simulink model "combined_1023"  (R2023a)
settings: Solver=ode45  StartTime=0  StopTime=20  FixedStep=0.001  RelTol=1e-3  AbsTol=1e-6
libraries: simulink x26, dspsigops x4, Solver_SF x1, slpidlib x1
settings Model: ExtModeTrigMode=oneshot  Creator=jhu  LastModifiedBy=Student
settings SolverCC: AutoScaleAbsTol=off  AlgebraicLoopSolver=TrustRegion
settings DataIOCC: SaveFormat=Array  SignalLoggingSaveFormat=ModelDataLogs  ReturnWorkspaceOutputs=off  SignalLoggingName=sigsOut
settings OptimizationCC: BlockReduction=off  BooleanDataType=off  ExpressionDepthLimit=2147483647  LifeSpan=inf
settings DebuggingCC: SaveWithParameterizedLinksMsg=none  UnderspecifiedInitializationDetection=Classic  MergeDetectMultiDrivingBlocksExec=none  SignalResolutionControl=TryResolveAllWithWarning  MultiTaskDSMMsg=warning  MultiTaskCondExecSysMsg=none  FcnCallInpInsideContextMsg=warning  UnconnectedInputMsg=warning  UnconnectedOutputMsg=warning  UnconnectedLineMsg=warning  StateNameClashWarn=warning  SFUnexpectedBacktrackingDiag=warning  SFNoUnconditionalDefaultTransitionDiag=warning  SFExecutionAtInitializationDiag=none  ArithmeticOperatorsInVariantConditions=warning
settings HardwareCC: ProdBitPerPointer=32  ProdBitPerSizeT=32  ProdBitPerPtrDiffT=32  ProdLargestAtomicFloat=None  ProdIntDivRoundTo=Undefined  ProdEndianess=Unspecified  ProdWordSize=32  ProdHWDeviceType=32-bit Generic  TargetUnknown=on
settings ModelReferenceCC: PropagateSignalLabelsOutOfModel=off
settings SFSimCC: SimUseLocalCustomCode=off  CustomCodeUndefinedFunction=UseInterfaceOnly
settings RTWCC: TemplateMakefile=grt_vc.tmf  RTWUseLocalCustomCode=off
settings CodeAppCC: StateflowObjectComments=on
settings GRTTargetCC: TargetFcnLib=ansi_tfl_tmw.mat  TargetLangStandard=C89/C90 (ANSI)  CombineOutputUpdateFcns=off  GRTInterface=on
settings ConfigComp: CovMetricSettings=dw  CovSaveCumulativeToWorkspaceVar=on  CovSaveSingleToWorkspaceVar=on  CovExternalEMLEnable=off

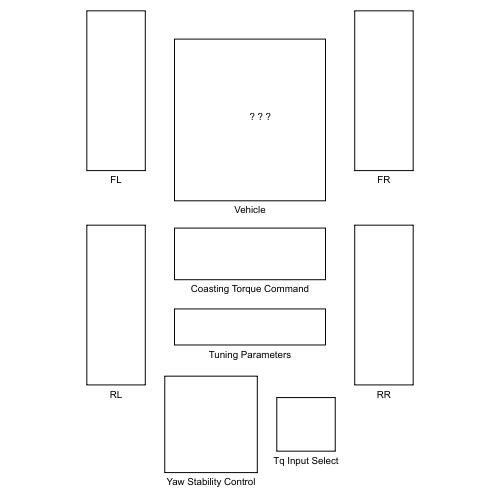
[thumbnail: Simulink's stored preview of the top-level diagram]
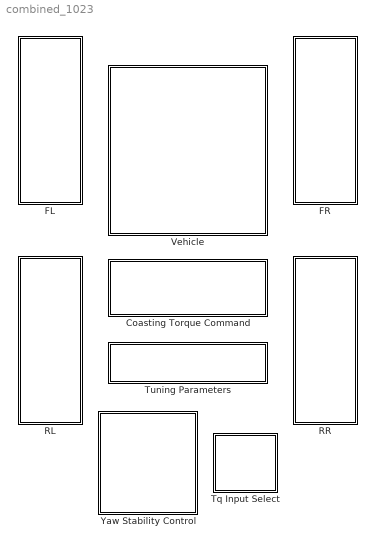
== system combined_1023 ==
  Coasting Torque Command : Subsystem
  FL : Subsystem
  FR : Subsystem
  RL : Subsystem
  RR : Subsystem
  Tq Input Select : Subsystem
  Tuning Parameters : Subsystem
  Vehicle : Subsystem
      mask Display: image('C:\Users\USER\Downloads\vehicle_icon.png'); % Use "Edit Image" on toolstrip to change.
  Yaw Stability Control : Subsystem

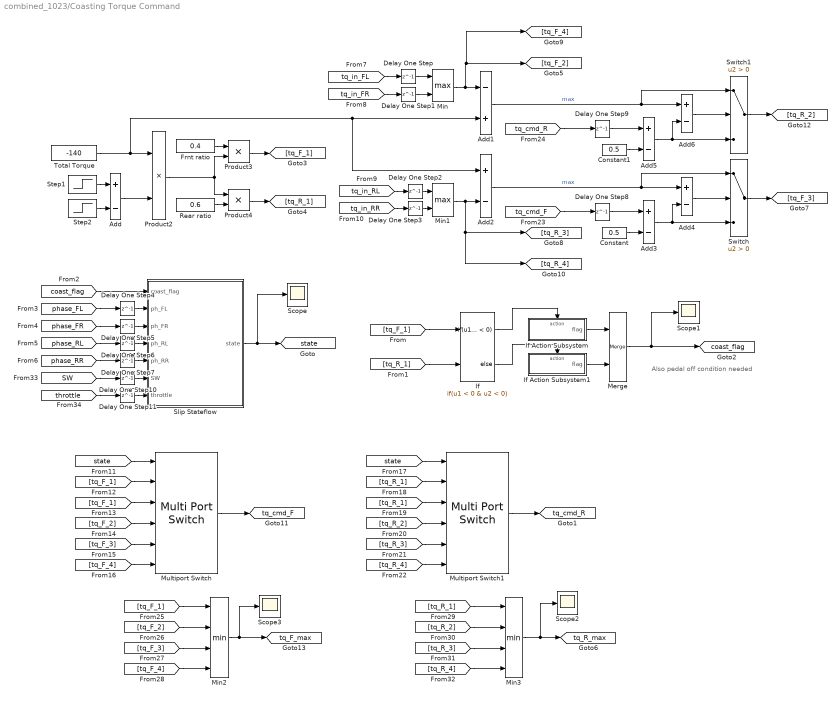
== system combined_1023/Coasting Torque Command ==
  note: Also pedal off condition needed
  Add{,2..6} (6 alike) : Sum  Inputs=+-
  Add1 : Sum  Inputs=-+
  Constant : Constant  Value=0.5
  Constant1 : Constant  Value=0.5
  Delay One Step{,1..7,10..11} (10 alike) : Delay  DelayLength=1
  Delay One Step8 : Delay  DelayLength=1  SampleTime=0.01
  Delay One Step9 : Delay  DelayLength=1  SampleTime=0.01
  Frnt ratio : Constant  Value=0.4  SampleTime=0.01
  If : If  NumInputs=2  IfExpression=u1 < 0 & u2 < 0
  If Action Subsystem : Subsystem  TreatAsAtomicUnit=on
  If Action Subsystem1 : Subsystem  TreatAsAtomicUnit=on
  Merge : Merge
  Min : MinMax  Function=max  Inputs=2
  Min1 : MinMax  Function=max  Inputs=2
  Min2 : MinMax  Inputs=4
  Min3 : MinMax  Inputs=4
  Multiport Switch : MultiPortSwitch  DataPortOrder=Zero-based contiguous  Inputs=5  zeroidx=on  SaturateOnIntegerOverflow=off  InputSameDT=off
  Multiport Switch1 : MultiPortSwitch  DataPortOrder=Zero-based contiguous  Inputs=5  zeroidx=on  SaturateOnIntegerOverflow=off  InputSameDT=off
  Product2 : Product
  Product3 : Product
  Product4 : Product
  Rear ratio : Constant  Value=0.6  SampleTime=0.01
  Scope{,1..3} (4 alike) : Scope
  Slip Stateflow : Stateflow chart  TreatAsAtomicUnit=on
  Step1 : Step  Time=5  SampleTime=0.01
  Step2 : Step  Time=20  SampleTime=0.01
  Switch : Switch  Criteria=u2 > Threshold  SaturateOnIntegerOverflow=off  InputSameDT=off
  Switch1 : Switch  Criteria=u2 > Threshold  SaturateOnIntegerOverflow=off  InputSameDT=off
  Total Torque : Constant  Value=-140  SampleTime=0.01
  tag scope: coast_flag=global, state=global, tq_F_max=global, tq_R_max=global, tq_cmd_F=global, tq_cmd_R=global
  wires:
  [tq_F_1] -> If/1
  [tq_R_1] -> If/2
  If/1 -> If Action Subsystem/Action
  If Action Subsystem/1(flag) -> Merge/1
  If Action Subsystem1/1(flag) -> Merge/2
  If/2 -> If Action Subsystem1/Action
  Merge/1 -> Scope1/1, [coast_flag]
  [coast_flag] -> Slip Stateflow/1(coast_flag)
  [phase_FL] -> Delay One Step4/1
  [phase_FR] -> Delay One Step5/1
  [phase_RL] -> Delay One Step6/1
  [phase_RR] -> Delay One Step7/1
  Slip Stateflow/1(state) -> Scope/1, [state]
  Step1/1 -> Add/1
  Step2/1 -> Add/2
  Add/1 -> Product2/2
  Product2/1 -> Product4/1, Product3/2
  Frnt ratio/1 -> Product3/1
  Rear ratio/1 -> Product4/2
  Product3/1 -> [tq_F_1]
  Product4/1 -> [tq_R_1]
  [tq_in_FL] -> Delay One Step/1
  [tq_in_FR] -> Delay One Step1/1
  Min/1 -> [tq_F_4], [tq_F_2], Add1/1
  [tq_in_RL] -> Delay One Step2/1
  [tq_in_RR] -> Delay One Step3/1
  Min1/1 -> [tq_R_4], [tq_R_3], Add2/2
  Add2/1 -> Switch/1, Add4/1  "max"
  [state] -> Multiport Switch/1
  [tq_F_1] -> Multiport Switch/2
  [tq_F_1] -> Multiport Switch/3
  [tq_F_2] -> Multiport Switch/4
  [tq_F_3] -> Multiport Switch/5
  [tq_F_4] -> Multiport Switch/6
  Multiport Switch/1 -> [tq_cmd_F]
  Multiport Switch1/1 -> [tq_cmd_R]
  [tq_R_3] -> Multiport Switch1/5
  [tq_R_4] -> Multiport Switch1/6
  [tq_R_2] -> Multiport Switch1/4
  [tq_R_1] -> Multiport Switch1/2
  [state] -> Multiport Switch1/1
  [tq_R_1] -> Multiport Switch1/3
  Delay One Step/1 -> Min/1
  Delay One Step1/1 -> Min/2
  Delay One Step2/1 -> Min1/1
  Delay One Step3/1 -> Min1/2
  Delay One Step4/1 -> Slip Stateflow/2(ph_FL)
  Delay One Step5/1 -> Slip Stateflow/3(ph_FR)
  Delay One Step6/1 -> Slip Stateflow/4(ph_RL)
  Delay One Step7/1 -> Slip Stateflow/5(ph_RR)
  [tq_cmd_F] -> Delay One Step8/1
  Delay One Step8/1 -> Add3/1
  Constant/1 -> Add3/2
  Add3/1 -> Add4/2, Switch/3
  Add4/1 -> Switch/2
  Switch/1 -> [tq_F_3]
  Switch1/1 -> [tq_R_2]
  Delay One Step9/1 -> Add5/1
  Add1/1 -> Switch1/1, Add6/1  "max"
  Add6/1 -> Switch1/2
  [tq_cmd_R] -> Delay One Step9/1
  Add5/1 -> Add6/2, Switch1/3
  Constant1/1 -> Add5/2
  Min2/1 -> Scope3/1, [tq_F_max]
  [tq_F_1] -> Min2/1
  [tq_F_2] -> Min2/2
  [tq_F_3] -> Min2/3
  [tq_F_4] -> Min2/4
  Min3/1 -> Scope2/1, [tq_R_max]
  [tq_R_1] -> Min3/1
  [tq_R_2] -> Min3/2
  [tq_R_3] -> Min3/3
  [tq_R_4] -> Min3/4
  [SW] -> Delay One Step10/1
  Delay One Step10/1 -> Slip Stateflow/6(SW)
  [throttle] -> Delay One Step11/1
  Delay One Step11/1 -> Slip Stateflow/7(throttle)
  Total Torque/1 -> Add2/1, Add1/2, Product2/1

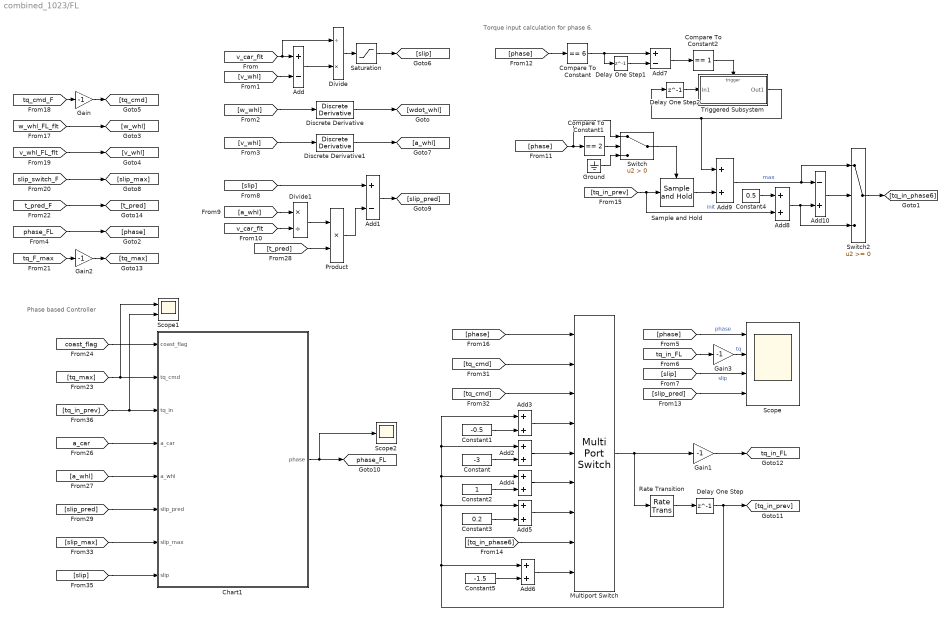
== system combined_1023/FL ==
  note: Phase based Controller
  note: Torque input calculation for phase 6.
  Add : Sum  Inputs=+-
  Add1 : Sum  Inputs=+-
  Add10 : Sum  Inputs=-+
  Add{2..6,8..9} (7 alike) : Sum
  Add7 : Sum  Inputs=+-
  Chart1 : Stateflow chart  TreatAsAtomicUnit=on
      settings: PortSchema="{\"entries\":[{\"content\":{\"sides\":[{\"content\":{\"connectorIds\":[\"In4\",\"In7\",\"In8\",\"In3\",\"In1\",\"In5\",\"In6\",\"In2\"]},\"type\":\"ConnectorPlacement.EquallySpacedRectSide\",\"uuid\":\"d1b40d47-5080-4bdb-9b64-2db0b8a6d570\"},{\"content\":{\"connectorIds\":[\"Out1\"],\"side\":\"RIGHT\"},\"type\":\"ConnectorPlacement.EquallySpacedRectSide\",\"uuid\":\"3562d231-244b-4945-a90c-51a654d62f0f\"},{\"content\":{\"side\":\"TOP\"},\"type\":\"ConnectorPlacement.EquallySpacedRectSide\",\"uuid\":\"6c914ffe-04dc-4ab2-bade-76d69248353c\"}]},\"type\":\"ConnectorPlacement.EquallySpacedConnector\",\"uuid\":\"36a59ec9-6bc3-461d-a020-c1da85e3b47f\"}],\"packageUris\":[\"http://schema.mathworks.com/mf0/Connector/R2020b\"],\"version\":\"1.0\"}"
  Compare To Constant : simulink/Logic and Bit Operations/Compare To Constant  relop===  const=6  OutDataTypeStr=boolean
  Compare To Constant1 : simulink/Logic and Bit Operations/Compare To Constant  relop===  const=2  OutDataTypeStr=boolean
  Compare To Constant2 : simulink/Logic and Bit Operations/Compare To Constant  relop===  const=1  OutDataTypeStr=boolean
  Constant : Constant  Value=-3
  Constant1 : Constant  Value=-0.5
  Constant2 : Constant
  Constant3 : Constant  Value=0.2
  Constant4 : Constant  Value=0.5  SampleTime=0.01
  Constant5 : Constant  Value=-1.5
  Delay One Step : Delay  DelayLength=1  SampleTime=0.01
  Delay One Step1 : Delay  DelayLength=1  SampleTime=0.01
  Delay One Step2 : Delay  DelayLength=1  InitialCondition=-1  SampleTime=0.01
  Discrete Derivative : simulink/Discrete/Discrete Derivative  gainval=1.0  ICPrevScaledInput=0.0  OutMin=[]  OutMax=[]  OutDataType=fixdt(1, 16)  OutScaling=2^-10  DoSatur=off
  Discrete Derivative1 : simulink/Discrete/Discrete Derivative  gainval=1.0  ICPrevScaledInput=0.0  OutMin=[]  OutMax=[]  OutDataType=fixdt(1, 16)  OutScaling=2^-10  DoSatur=off
  Divide : Product  Inputs=/*
  Divide1 : Product  Inputs=*/
  Gain{,1..3} (4 alike) : Gain  Gain=-1
  Ground : Ground
  Multiport Switch : MultiPortSwitch  DataPortOrder=Zero-based contiguous  Inputs=8  zeroidx=on  SaturateOnIntegerOverflow=off  InputSameDT=off
  Product : Product
  Rate Transition : RateTransition  OutPortSampleTime=0.01
  Sample and Hold : dspsigops/Sample and Hold  trig=Rising edge  initCond=0  latchinput=off
  Saturation : Saturate  UpperLimit=1  LowerLimit=-1
  Scope : Scope  NumInputPorts=4
  Scope1 : Scope  NumInputPorts=2
  Scope2 : Scope
  Switch : Switch  Criteria=u2 > Threshold  SaturateOnIntegerOverflow=off  InputSameDT=off
  Switch2 : Switch  SaturateOnIntegerOverflow=off  InputSameDT=off
  Triggered Subsystem : Subsystem  TreatAsAtomicUnit=on
  tag scope: phase_FL=global, tq_in_FL=global
  wires:
  [v_car_flt] -> Divide/1, Add/1
  [v_whl] -> Add/2
  Add/1 -> Divide/2
  Divide/1 -> Saturation/1
  Saturation/1 -> [slip]
  [w_whl] -> Discrete Derivative/1
  Discrete Derivative/1 -> [wdot_whl]
  [v_whl] -> Discrete Derivative1/1
  Discrete Derivative1/1 -> [a_whl]
  [slip_switch_F] -> [slip_max]
  [w_whl_FL_flt] -> [w_whl]
  [v_whl_FL_flt] -> [v_whl]
  [phase] -> Multiport Switch/1
  [tq_cmd] -> Multiport Switch/2
  [tq_cmd] -> Multiport Switch/3
  Rate Transition/1 -> Delay One Step/1
  Multiport Switch/1 -> Gain1/1, Rate Transition/1
  [slip] -> Add1/1
  [a_whl] -> Divide1/1
  [v_car_flt] -> Divide1/2
  Divide1/1 -> Product/1
  Add1/1 -> [slip_pred]
  [t_pred_F] -> [t_pred]
  [t_pred] -> Product/2
  Product/1 -> Add1/2
  Add2/1 -> Multiport Switch/5
  Constant/1 -> Add2/2
  Constant1/1 -> Add3/2
  Add3/1 -> Multiport Switch/4
  Gain/1 -> [tq_cmd]
  Gain1/1 -> [tq_in_FL]
  Add4/1 -> Multiport Switch/6
  Constant2/1 -> Add4/2
  Constant3/1 -> Add5/2
  Add5/1 -> Multiport Switch/7
  Ground/1 -> Switch/3
  Switch/1 -> Sample and Hold/Trigger
  Sample and Hold/1 -> Add9/2
  [phase] -> Compare To Constant/1
  Compare To Constant/1 -> Delay One Step1/1, Add7/1
  Delay One Step1/1 -> Add7/2
  Add7/1 -> Compare To Constant2/1
  [phase] -> Switch/1, Compare To Constant1/1
  Compare To Constant1/1 -> Switch/2
  Compare To Constant2/1 -> Triggered Subsystem/Trigger
  Constant5/1 -> Add6/2
  Add6/1 -> Multiport Switch/9
  Delay One Step/1 -> [tq_in_prev], Add3/1, Add2/1, Add4/1, Add5/1, Add6/1
  Triggered Subsystem/1(Out1) -> Add9/1, Delay One Step2/1
  Delay One Step2/1 -> Triggered Subsystem/1(In1)
  [tq_in_prev] -> Add8/2, Sample and Hold/1  "init"
  [phase] -> Scope/1  "phase"
  [tq_in_FL] -> Gain3/1
  Gain3/1 -> Scope/2  "tq"
  [slip] -> Scope/3  "slip"
  Add9/1 -> Switch2/1, Add10/1  "max"
  Constant4/1 -> Add8/1
  Add8/1 -> Switch2/3, Add10/2
  Add10/1 -> Switch2/2
  Switch2/1 -> [tq_in_phase6]
  [slip_pred] -> Scope/4
  [tq_in_phase6] -> Multiport Switch/8
  [phase_FL] -> [phase]
  [tq_in_prev] -> Scope1/2, Chart1/8(tq_in)
  [a_whl] -> Chart1/1(a_whl)
  [slip] -> Chart1/2(slip)
  [slip_pred] -> Chart1/5(slip_pred)
  [slip_max] -> Chart1/6(slip_max)
  [coast_flag] -> Chart1/4(coast_flag)
  Chart1/1(phase) -> Scope2/1, [phase_FL]
  [a_car] -> Chart1/3(a_car)
  [tq_max] -> Scope1/1, Chart1/7(tq_cmd)
  [tq_cmd_F] -> Gain/1
  Gain2/1 -> [tq_max]
  [tq_F_max] -> Gain2/1

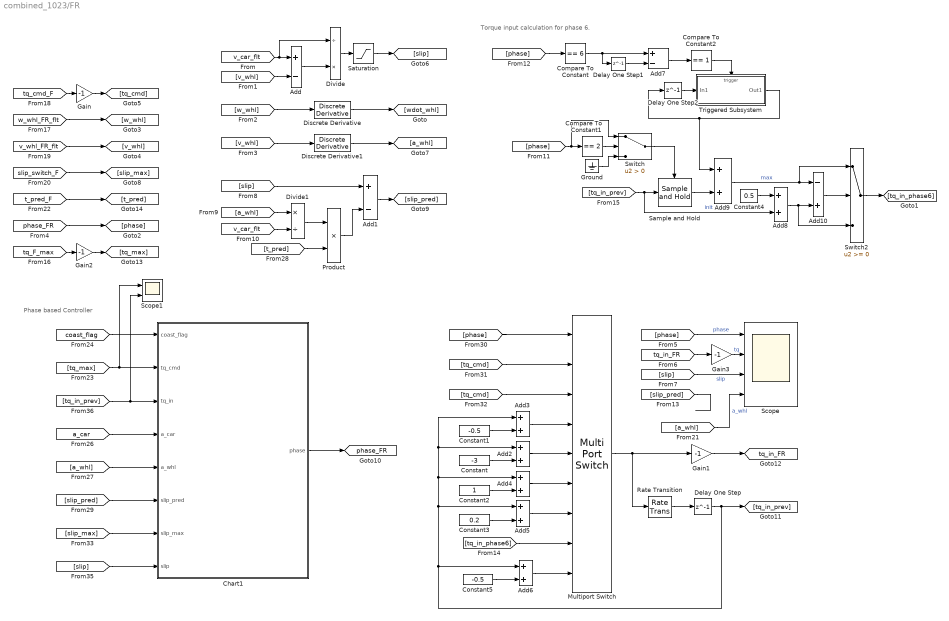
== system combined_1023/FR ==
  note: Phase based Controller
  note: Torque input calculation for phase 6.
  Add : Sum  Inputs=+-
  Add1 : Sum  Inputs=+-
  Add10 : Sum  Inputs=-+
  Add{2..6,8..9} (7 alike) : Sum
  Add7 : Sum  Inputs=+-
  Chart1 : Stateflow chart  TreatAsAtomicUnit=on
      settings: PortSchema="{\"entries\":[{\"content\":{\"sides\":[{\"content\":{\"connectorIds\":[\"In4\",\"In7\",\"In8\",\"In3\",\"In1\",\"In5\",\"In6\",\"In2\"]},\"type\":\"ConnectorPlacement.EquallySpacedRectSide\",\"uuid\":\"d1b40d47-5080-4bdb-9b64-2db0b8a6d570\"},{\"content\":{\"connectorIds\":[\"Out1\"],\"side\":\"RIGHT\"},\"type\":\"ConnectorPlacement.EquallySpacedRectSide\",\"uuid\":\"3562d231-244b-4945-a90c-51a654d62f0f\"},{\"content\":{\"side\":\"TOP\"},\"type\":\"ConnectorPlacement.EquallySpacedRectSide\",\"uuid\":\"6c914ffe-04dc-4ab2-bade-76d69248353c\"}]},\"type\":\"ConnectorPlacement.EquallySpacedConnector\",\"uuid\":\"36a59ec9-6bc3-461d-a020-c1da85e3b47f\"}],\"packageUris\":[\"http://schema.mathworks.com/mf0/Connector/R2020b\"],\"version\":\"1.0\"}"
  Compare To Constant : simulink/Logic and Bit Operations/Compare To Constant  relop===  const=6  OutDataTypeStr=boolean
  Compare To Constant1 : simulink/Logic and Bit Operations/Compare To Constant  relop===  const=2  OutDataTypeStr=boolean
  Compare To Constant2 : simulink/Logic and Bit Operations/Compare To Constant  relop===  const=1  OutDataTypeStr=boolean
  Constant : Constant  Value=-3
  Constant1 : Constant  Value=-0.5
  Constant2 : Constant
  Constant3 : Constant  Value=0.2
  Constant4 : Constant  Value=0.5  SampleTime=0.01
  Constant5 : Constant  Value=-0.5
  Delay One Step : Delay  DelayLength=1  SampleTime=0.01
  Delay One Step1 : Delay  DelayLength=1  SampleTime=0.01
  Delay One Step2 : Delay  DelayLength=1  InitialCondition=-1  SampleTime=0.01
  Discrete Derivative : simulink/Discrete/Discrete Derivative  gainval=1.0  ICPrevScaledInput=0.0  OutMin=[]  OutMax=[]  OutDataType=fixdt(1, 16)  OutScaling=2^-10  DoSatur=off
  Discrete Derivative1 : simulink/Discrete/Discrete Derivative  gainval=1.0  ICPrevScaledInput=0.0  OutMin=[]  OutMax=[]  OutDataType=fixdt(1, 16)  OutScaling=2^-10  DoSatur=off
  Divide : Product  Inputs=/*
  Divide1 : Product  Inputs=*/
  Gain{,1..3} (4 alike) : Gain  Gain=-1
  Ground : Ground
  Multiport Switch : MultiPortSwitch  DataPortOrder=Zero-based contiguous  Inputs=8  zeroidx=on  SaturateOnIntegerOverflow=off  InputSameDT=off
  Product : Product
  Rate Transition : RateTransition  OutPortSampleTime=0.01
  Sample and Hold : dspsigops/Sample and Hold  trig=Rising edge  initCond=0  latchinput=off
  Saturation : Saturate  UpperLimit=1  LowerLimit=-1
  Scope : Scope  NumInputPorts=4
  Scope1 : Scope  NumInputPorts=2
  Switch : Switch  Criteria=u2 > Threshold  SaturateOnIntegerOverflow=off  InputSameDT=off
  Switch2 : Switch  SaturateOnIntegerOverflow=off  InputSameDT=off
  Triggered Subsystem : Subsystem  TreatAsAtomicUnit=on
  tag scope: phase_FR=global, tq_in_FR=global
  wires:
  [v_car_flt] -> Divide/1, Add/1
  [v_whl] -> Add/2
  Add/1 -> Divide/2
  Divide/1 -> Saturation/1
  Saturation/1 -> [slip]
  [w_whl] -> Discrete Derivative/1
  Discrete Derivative/1 -> [wdot_whl]
  [v_whl] -> Discrete Derivative1/1
  Discrete Derivative1/1 -> [a_whl]
  [slip_switch_F] -> [slip_max]
  [w_whl_FR_flt] -> [w_whl]
  [v_whl_FR_flt] -> [v_whl]
  [phase] -> Multiport Switch/1
  [tq_cmd] -> Multiport Switch/2
  [tq_cmd] -> Multiport Switch/3
  Rate Transition/1 -> Delay One Step/1
  Multiport Switch/1 -> Gain1/1, Rate Transition/1
  [slip] -> Add1/1
  [a_whl] -> Divide1/1
  [v_car_flt] -> Divide1/2
  Divide1/1 -> Product/1
  Add1/1 -> [slip_pred]
  [t_pred_F] -> [t_pred]
  [t_pred] -> Product/2
  Product/1 -> Add1/2
  Add2/1 -> Multiport Switch/5
  Constant/1 -> Add2/2
  Constant1/1 -> Add3/2
  Add3/1 -> Multiport Switch/4
  Gain/1 -> [tq_cmd]
  Gain1/1 -> [tq_in_FR]
  Add4/1 -> Multiport Switch/6
  Constant2/1 -> Add4/2
  Constant3/1 -> Add5/2
  Add5/1 -> Multiport Switch/7
  Ground/1 -> Switch/3
  Switch/1 -> Sample and Hold/Trigger
  Sample and Hold/1 -> Add9/2
  [phase] -> Compare To Constant/1
  Compare To Constant/1 -> Delay One Step1/1, Add7/1
  Delay One Step1/1 -> Add7/2
  Add7/1 -> Compare To Constant2/1
  [phase] -> Switch/1, Compare To Constant1/1
  Compare To Constant1/1 -> Switch/2
  Compare To Constant2/1 -> Triggered Subsystem/Trigger
  Constant5/1 -> Add6/2
  Add6/1 -> Multiport Switch/9
  Delay One Step/1 -> [tq_in_prev], Add3/1, Add2/1, Add4/1, Add5/1, Add6/1
  Triggered Subsystem/1(Out1) -> Add9/1, Delay One Step2/1
  Delay One Step2/1 -> Triggered Subsystem/1(In1)
  [tq_in_prev] -> Add8/2, Sample and Hold/1  "init"
  [tq_max] -> Scope1/1, Chart1/7(tq_cmd)
  [coast_flag] -> Chart1/4(coast_flag)
  Chart1/1(phase) -> [phase_FR]
  [a_car] -> Chart1/3(a_car)
  [a_whl] -> Chart1/1(a_whl)
  [slip_pred] -> Chart1/5(slip_pred)
  [slip_max] -> Chart1/6(slip_max)
  [slip] -> Chart1/2(slip)
  [tq_in_prev] -> Scope1/2, Chart1/8(tq_in)
  [phase] -> Scope/1  "phase"
  [tq_in_FR] -> Gain3/1
  Gain3/1 -> Scope/2  "tq"
  [slip] -> Scope/3  "slip"
  Add9/1 -> Switch2/1, Add10/1  "max"
  Constant4/1 -> Add8/1
  Add8/1 -> Switch2/3, Add10/2
  Add10/1 -> Switch2/2
  Switch2/1 -> [tq_in_phase6]
  [slip_pred] -> ?
  [tq_in_phase6] -> Multiport Switch/8
  [phase_FR] -> [phase]
  [tq_cmd_F] -> Gain/1
  [tq_F_max] -> Gain2/1
  Gain2/1 -> [tq_max]
  [a_whl] -> Scope/4  "a_whl"

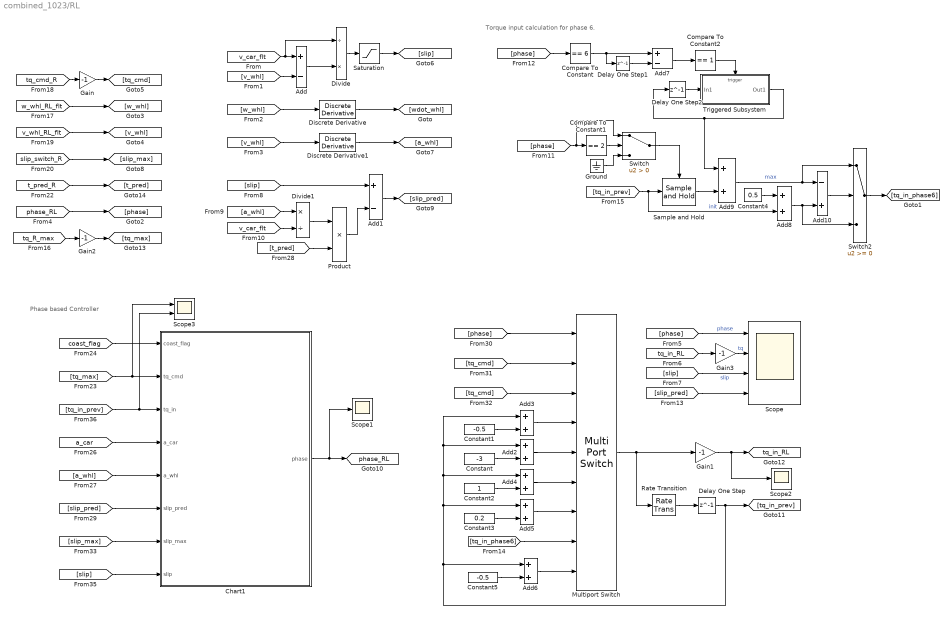
== system combined_1023/RL ==
  note: Torque input calculation for phase 6.
  note: Phase based Controller
  Add : Sum  Inputs=+-
  Add1 : Sum  Inputs=+-
  Add10 : Sum  Inputs=-+
  Add{2..6,8..9} (7 alike) : Sum
  Add7 : Sum  Inputs=+-
  Chart1 : Stateflow chart  TreatAsAtomicUnit=on
      settings: PortSchema="{\"entries\":[{\"content\":{\"sides\":[{\"content\":{\"connectorIds\":[\"In4\",\"In7\",\"In8\",\"In3\",\"In1\",\"In5\",\"In6\",\"In2\"]},\"type\":\"ConnectorPlacement.EquallySpacedRectSide\",\"uuid\":\"d1b40d47-5080-4bdb-9b64-2db0b8a6d570\"},{\"content\":{\"connectorIds\":[\"Out1\"],\"side\":\"RIGHT\"},\"type\":\"ConnectorPlacement.EquallySpacedRectSide\",\"uuid\":\"3562d231-244b-4945-a90c-51a654d62f0f\"},{\"content\":{\"side\":\"TOP\"},\"type\":\"ConnectorPlacement.EquallySpacedRectSide\",\"uuid\":\"6c914ffe-04dc-4ab2-bade-76d69248353c\"}]},\"type\":\"ConnectorPlacement.EquallySpacedConnector\",\"uuid\":\"36a59ec9-6bc3-461d-a020-c1da85e3b47f\"}],\"packageUris\":[\"http://schema.mathworks.com/mf0/Connector/R2020b\"],\"version\":\"1.0\"}"
  Compare To Constant : simulink/Logic and Bit Operations/Compare To Constant  relop===  const=6  OutDataTypeStr=boolean
  Compare To Constant1 : simulink/Logic and Bit Operations/Compare To Constant  relop===  const=2  OutDataTypeStr=boolean
  Compare To Constant2 : simulink/Logic and Bit Operations/Compare To Constant  relop===  const=1  OutDataTypeStr=boolean
  Constant : Constant  Value=-3
  Constant1 : Constant  Value=-0.5
  Constant2 : Constant
  Constant3 : Constant  Value=0.2
  Constant4 : Constant  Value=0.5  SampleTime=0.01
  Constant5 : Constant  Value=-0.5
  Delay One Step : Delay  DelayLength=1  SampleTime=0.01
  Delay One Step1 : Delay  DelayLength=1  SampleTime=0.01
  Delay One Step2 : Delay  DelayLength=1  InitialCondition=-1  SampleTime=0.01
  Discrete Derivative : simulink/Discrete/Discrete Derivative  gainval=1.0  ICPrevScaledInput=0.0  OutMin=[]  OutMax=[]  OutDataType=fixdt(1, 16)  OutScaling=2^-10  DoSatur=off
  Discrete Derivative1 : simulink/Discrete/Discrete Derivative  gainval=1.0  ICPrevScaledInput=0.0  OutMin=[]  OutMax=[]  OutDataType=fixdt(1, 16)  OutScaling=2^-10  DoSatur=off
  Divide : Product  Inputs=/*
  Divide1 : Product  Inputs=*/
  Gain{,1..3} (4 alike) : Gain  Gain=-1
  Ground : Ground
  Multiport Switch : MultiPortSwitch  DataPortOrder=Zero-based contiguous  Inputs=8  zeroidx=on  SaturateOnIntegerOverflow=off  InputSameDT=off
  Product : Product
  Rate Transition : RateTransition  OutPortSampleTime=0.01
  Sample and Hold : dspsigops/Sample and Hold  trig=Rising edge  initCond=0  latchinput=off
  Saturation : Saturate  UpperLimit=1  LowerLimit=-1
  Scope : Scope  NumInputPorts=4
  Scope1 : Scope
  Scope2 : Scope
  Scope3 : Scope  NumInputPorts=2
  Switch : Switch  Criteria=u2 > Threshold  SaturateOnIntegerOverflow=off  InputSameDT=off
  Switch2 : Switch  SaturateOnIntegerOverflow=off  InputSameDT=off
  Triggered Subsystem : Subsystem  TreatAsAtomicUnit=on
  tag scope: phase_RL=global, tq_in_RL=global
  wires:
  [tq_in_phase6] -> Multiport Switch/8
  [slip_pred] -> Scope/4
  Switch2/1 -> [tq_in_phase6]
  Add10/1 -> Switch2/2
  Add8/1 -> Add10/2, Switch2/3
  Constant4/1 -> Add8/1
  Add9/1 -> Add10/1, Switch2/1  "max"
  [slip] -> Scope/3  "slip"
  Gain3/1 -> Scope/2  "tq"
  [tq_in_RL] -> Gain3/1
  [phase] -> Scope/1  "phase"
  [tq_in_prev] -> Sample and Hold/1, Add8/2  "init"
  Delay One Step2/1 -> Triggered Subsystem/1(In1)
  Triggered Subsystem/1(Out1) -> Delay One Step2/1, Add9/1
  Delay One Step/1 -> Add6/1, Add5/1, Add4/1, Add2/1, Add3/1, [tq_in_prev]
  Add6/1 -> Multiport Switch/9
  Constant5/1 -> Add6/2
  Compare To Constant2/1 -> Triggered Subsystem/Trigger
  Compare To Constant1/1 -> Switch/2
  [phase] -> Compare To Constant1/1, Switch/1
  Add7/1 -> Compare To Constant2/1
  Delay One Step1/1 -> Add7/2
  Compare To Constant/1 -> Add7/1, Delay One Step1/1
  [phase] -> Compare To Constant/1
  Sample and Hold/1 -> Add9/2
  Switch/1 -> Sample and Hold/Trigger
  Ground/1 -> Switch/3
  Add5/1 -> Multiport Switch/7
  Constant3/1 -> Add5/2
  Constant2/1 -> Add4/2
  Add4/1 -> Multiport Switch/6
  Gain1/1 -> Scope2/1, [tq_in_RL]
  Gain/1 -> [tq_cmd]
  Add3/1 -> Multiport Switch/4
  Constant1/1 -> Add3/2
  Constant/1 -> Add2/2
  Add2/1 -> Multiport Switch/5
  Product/1 -> Add1/2
  [t_pred] -> Product/2
  [t_pred_R] -> [t_pred]
  Add1/1 -> [slip_pred]
  Divide1/1 -> Product/1
  [v_car_flt] -> Divide1/2
  [a_whl] -> Divide1/1
  [slip] -> Add1/1
  Multiport Switch/1 -> Rate Transition/1, Gain1/1
  Rate Transition/1 -> Delay One Step/1
  [tq_cmd] -> Multiport Switch/3
  [tq_cmd] -> Multiport Switch/2
  [phase] -> Multiport Switch/1
  [v_whl_RL_flt] -> [v_whl]
  [w_whl_RL_flt] -> [w_whl]
  [slip_switch_R] -> [slip_max]
  Discrete Derivative1/1 -> [a_whl]
  [v_whl] -> Discrete Derivative1/1
  Discrete Derivative/1 -> [wdot_whl]
  [w_whl] -> Discrete Derivative/1
  Saturation/1 -> [slip]
  Divide/1 -> Saturation/1
  Add/1 -> Divide/2
  [v_whl] -> Add/2
  [v_car_flt] -> Add/1, Divide/1
  [phase_RL] -> [phase]
  [tq_in_prev] -> Scope3/2, Chart1/8(tq_in)
  [a_whl] -> Chart1/1(a_whl)
  [slip] -> Chart1/2(slip)
  [slip_pred] -> Chart1/5(slip_pred)
  [slip_max] -> Chart1/6(slip_max)
  [coast_flag] -> Chart1/4(coast_flag)
  Chart1/1(phase) -> Scope1/1, [phase_RL]
  [a_car] -> Chart1/3(a_car)
  [tq_max] -> Scope3/1, Chart1/7(tq_cmd)
  [tq_cmd_R] -> Gain/1
  [tq_R_max] -> Gain2/1
  Gain2/1 -> [tq_max]

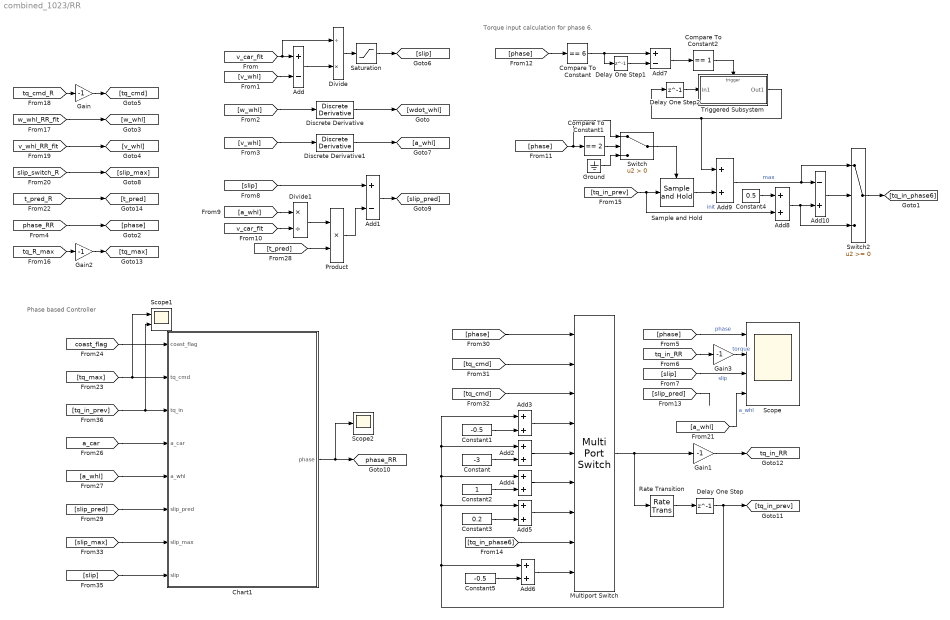
== system combined_1023/RR ==
  note: Phase based Controller
  note: Torque input calculation for phase 6.
  Add : Sum  Inputs=+-
  Add1 : Sum  Inputs=+-
  Add10 : Sum  Inputs=-+
  Add{2..6,8..9} (7 alike) : Sum
  Add7 : Sum  Inputs=+-
  Chart1 : Stateflow chart  TreatAsAtomicUnit=on
      settings: PortSchema="{\"entries\":[{\"content\":{\"sides\":[{\"content\":{\"connectorIds\":[\"In4\",\"In7\",\"In8\",\"In3\",\"In1\",\"In5\",\"In6\",\"In2\"]},\"type\":\"ConnectorPlacement.EquallySpacedRectSide\",\"uuid\":\"d1b40d47-5080-4bdb-9b64-2db0b8a6d570\"},{\"content\":{\"connectorIds\":[\"Out1\"],\"side\":\"RIGHT\"},\"type\":\"ConnectorPlacement.EquallySpacedRectSide\",\"uuid\":\"3562d231-244b-4945-a90c-51a654d62f0f\"},{\"content\":{\"side\":\"TOP\"},\"type\":\"ConnectorPlacement.EquallySpacedRectSide\",\"uuid\":\"6c914ffe-04dc-4ab2-bade-76d69248353c\"}]},\"type\":\"ConnectorPlacement.EquallySpacedConnector\",\"uuid\":\"36a59ec9-6bc3-461d-a020-c1da85e3b47f\"}],\"packageUris\":[\"http://schema.mathworks.com/mf0/Connector/R2020b\"],\"version\":\"1.0\"}"
  Compare To Constant : simulink/Logic and Bit Operations/Compare To Constant  relop===  const=6  OutDataTypeStr=boolean
  Compare To Constant1 : simulink/Logic and Bit Operations/Compare To Constant  relop===  const=2  OutDataTypeStr=boolean
  Compare To Constant2 : simulink/Logic and Bit Operations/Compare To Constant  relop===  const=1  OutDataTypeStr=boolean
  Constant : Constant  Value=-3
  Constant1 : Constant  Value=-0.5
  Constant2 : Constant
  Constant3 : Constant  Value=0.2
  Constant4 : Constant  Value=0.5  SampleTime=0.01
  Constant5 : Constant  Value=-0.5
  Delay One Step : Delay  DelayLength=1  SampleTime=0.01
  Delay One Step1 : Delay  DelayLength=1  SampleTime=0.01
  Delay One Step2 : Delay  DelayLength=1  InitialCondition=-1  SampleTime=0.01
  Discrete Derivative : simulink/Discrete/Discrete Derivative  gainval=1.0  ICPrevScaledInput=0.0  OutMin=[]  OutMax=[]  OutDataType=fixdt(1, 16)  OutScaling=2^-10  DoSatur=off
  Discrete Derivative1 : simulink/Discrete/Discrete Derivative  gainval=1.0  ICPrevScaledInput=0.0  OutMin=[]  OutMax=[]  OutDataType=fixdt(1, 16)  OutScaling=2^-10  DoSatur=off
  Divide : Product  Inputs=/*
  Divide1 : Product  Inputs=*/
  Gain{,1..3} (4 alike) : Gain  Gain=-1
  Ground : Ground
  Multiport Switch : MultiPortSwitch  DataPortOrder=Zero-based contiguous  Inputs=8  zeroidx=on  SaturateOnIntegerOverflow=off  InputSameDT=off
  Product : Product
  Rate Transition : RateTransition  OutPortSampleTime=0.01
  Sample and Hold : dspsigops/Sample and Hold  trig=Rising edge  initCond=0  latchinput=off
  Saturation : Saturate  UpperLimit=1  LowerLimit=-1
  Scope : Scope  NumInputPorts=4
  Scope1 : Scope  NumInputPorts=2
  Scope2 : Scope
  Switch : Switch  Criteria=u2 > Threshold  SaturateOnIntegerOverflow=off  InputSameDT=off
  Switch2 : Switch  SaturateOnIntegerOverflow=off  InputSameDT=off
  Triggered Subsystem : Subsystem  TreatAsAtomicUnit=on
  tag scope: phase_RR=global, tq_in_RR=global
  wires:
  [v_car_flt] -> Divide/1, Add/1
  [v_whl] -> Add/2
  Add/1 -> Divide/2
  Divide/1 -> Saturation/1
  Saturation/1 -> [slip]
  [w_whl] -> Discrete Derivative/1
  Discrete Derivative/1 -> [wdot_whl]
  [v_whl] -> Discrete Derivative1/1
  Discrete Derivative1/1 -> [a_whl]
  [slip_switch_R] -> [slip_max]
  [w_whl_RR_flt] -> [w_whl]
  [v_whl_RR_flt] -> [v_whl]
  [tq_cmd_R] -> Gain/1
  [phase] -> Multiport Switch/1
  [tq_cmd] -> Multiport Switch/2
  [tq_cmd] -> Multiport Switch/3
  Rate Transition/1 -> Delay One Step/1
  Multiport Switch/1 -> Gain1/1, Rate Transition/1
  [slip] -> Add1/1
  [a_whl] -> Divide1/1
  [v_car_flt] -> Divide1/2
  Divide1/1 -> Product/1
  Add1/1 -> [slip_pred]
  [t_pred_R] -> [t_pred]
  [t_pred] -> Product/2
  Product/1 -> Add1/2
  Add2/1 -> Multiport Switch/5
  Constant/1 -> Add2/2
  Constant1/1 -> Add3/2
  Add3/1 -> Multiport Switch/4
  Gain/1 -> [tq_cmd]
  Gain1/1 -> [tq_in_RR]
  Add4/1 -> Multiport Switch/6
  Constant2/1 -> Add4/2
  Constant3/1 -> Add5/2
  Add5/1 -> Multiport Switch/7
  Ground/1 -> Switch/3
  Switch/1 -> Sample and Hold/Trigger
  Sample and Hold/1 -> Add9/2
  [phase] -> Compare To Constant/1
  Compare To Constant/1 -> Delay One Step1/1, Add7/1
  Delay One Step1/1 -> Add7/2
  Add7/1 -> Compare To Constant2/1
  [phase] -> Switch/1, Compare To Constant1/1
  Compare To Constant1/1 -> Switch/2
  Compare To Constant2/1 -> Triggered Subsystem/Trigger
  Constant5/1 -> Add6/2
  Add6/1 -> Multiport Switch/9
  Delay One Step/1 -> [tq_in_prev], Add3/1, Add2/1, Add4/1, Add5/1, Add6/1
  Triggered Subsystem/1(Out1) -> Add9/1, Delay One Step2/1
  Delay One Step2/1 -> Triggered Subsystem/1(In1)
  [tq_in_prev] -> Add8/2, Sample and Hold/1  "init"
  [phase] -> Scope/1  "phase"
  [tq_in_RR] -> Gain3/1
  Gain3/1 -> Scope/2  "torque"
  [slip] -> Scope/3  "slip"
  Add9/1 -> Switch2/1, Add10/1  "max"
  Constant4/1 -> Add8/1
  Add8/1 -> Switch2/3, Add10/2
  Add10/1 -> Switch2/2
  Switch2/1 -> [tq_in_phase6]
  [slip_pred] -> ?
  [tq_in_phase6] -> Multiport Switch/8
  [phase_RR] -> [phase]
  [tq_in_prev] -> Scope1/2, Chart1/8(tq_in)
  [a_whl] -> Chart1/1(a_whl)
  [slip] -> Chart1/2(slip)
  [slip_pred] -> Chart1/5(slip_pred)
  [slip_max] -> Chart1/6(slip_max)
  [coast_flag] -> Chart1/4(coast_flag)
  Chart1/1(phase) -> Scope2/1, [phase_RR]
  [a_car] -> Chart1/3(a_car)
  [tq_max] -> Scope1/1, Chart1/7(tq_cmd)
  Gain2/1 -> [tq_max]
  [tq_R_max] -> Gain2/1
  [a_whl] -> Scope/4  "a_whl"

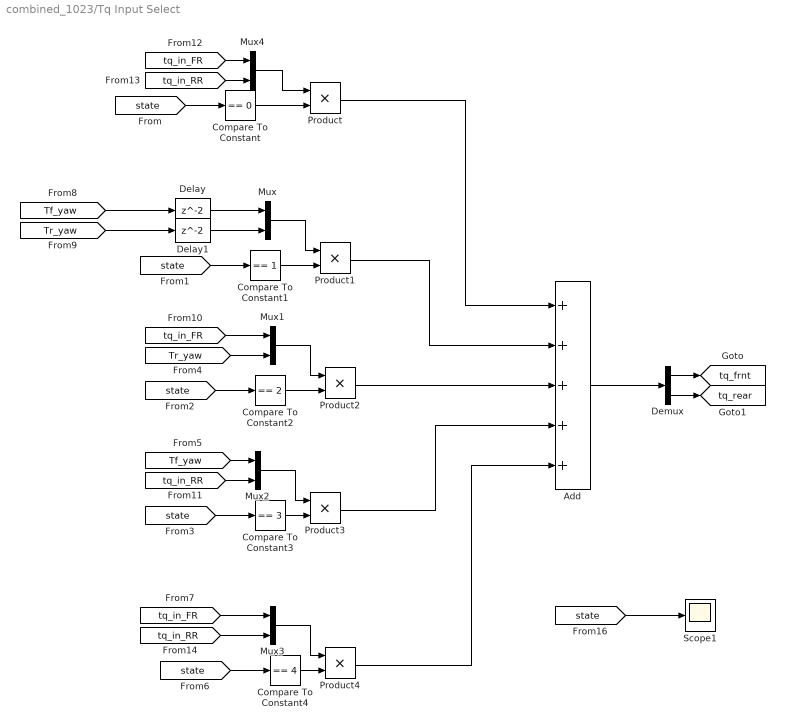
== system combined_1023/Tq Input Select ==
  Add : Sum  Inputs=+++++
  Compare To Constant : simulink/Logic and Bit Operations/Compare To Constant  relop===  const=0  OutDataTypeStr=boolean
  Compare To Constant1 : simulink/Logic and Bit Operations/Compare To Constant  relop===  const=1  OutDataTypeStr=boolean
  Compare To Constant2 : simulink/Logic and Bit Operations/Compare To Constant  relop===  const=2  OutDataTypeStr=boolean
  Compare To Constant3 : simulink/Logic and Bit Operations/Compare To Constant  relop===  const=3  OutDataTypeStr=boolean
  Compare To Constant4 : simulink/Logic and Bit Operations/Compare To Constant  relop===  const=4  OutDataTypeStr=boolean
  Delay : Delay
  Delay1 : Delay
  Demux : Demux  Outputs=2
  Mux{,1..4} (5 alike) : Mux  Inputs=2
  Product{,1..4} (5 alike) : Product
  Scope1 : Scope
  tag scope: tq_frnt=global, tq_rear=global
  wires:
  [state] -> Compare To Constant/1
  [state] -> Compare To Constant1/1
  [state] -> Compare To Constant2/1
  [state] -> Compare To Constant3/1
  Compare To Constant3/1 -> Product3/2
  Compare To Constant1/1 -> Product1/2
  Compare To Constant/1 -> Product/2
  Product/1 -> Add/1
  Mux/1 -> Product1/1
  [Tf_yaw] -> Delay/1
  [Tr_yaw] -> Delay1/1
  Mux1/1 -> Product2/1
  Compare To Constant2/1 -> Product2/2
  [Tr_yaw] -> Mux1/2
  Mux2/1 -> Product3/1
  [Tf_yaw] -> Mux2/1
  Compare To Constant4/1 -> Product4/2
  Mux3/1 -> Product4/1
  [state] -> Compare To Constant4/1
  Product1/1 -> Add/2
  Product2/1 -> Add/3
  Product3/1 -> Add/4
  Product4/1 -> Add/5
  [tq_in_FR] -> Mux1/1
  [tq_in_RR] -> Mux2/2
  Add/1 -> Demux/1
  Demux/1 -> [tq_frnt]
  Demux/2 -> [tq_rear]
  [tq_in_FR] -> Mux3/1
  [tq_in_RR] -> Mux3/2
  [state] -> Scope1/1
  [tq_in_FR] -> Mux4/1
  [tq_in_RR] -> Mux4/2
  Mux4/1 -> Product/1
  Delay/1 -> Mux/1
  Delay1/1 -> Mux/2

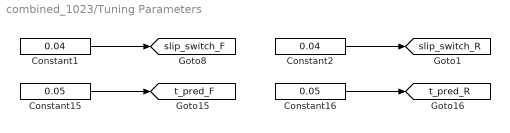
== system combined_1023/Tuning Parameters ==
  Constant1 : Constant  Value=0.04  SampleTime=0.01
  Constant15 : Constant  Value=0.05  SampleTime=0.01
  Constant16 : Constant  Value=0.05  SampleTime=0.01
  Constant2 : Constant  Value=0.04  SampleTime=0.01
  tag scope: slip_switch_F=global, slip_switch_R=global, t_pred_F=global, t_pred_R=global
  wires:
  Constant1/1 -> [slip_switch_F]
  Constant2/1 -> [slip_switch_R]
  Constant15/1 -> [t_pred_F]
  Constant16/1 -> [t_pred_R]

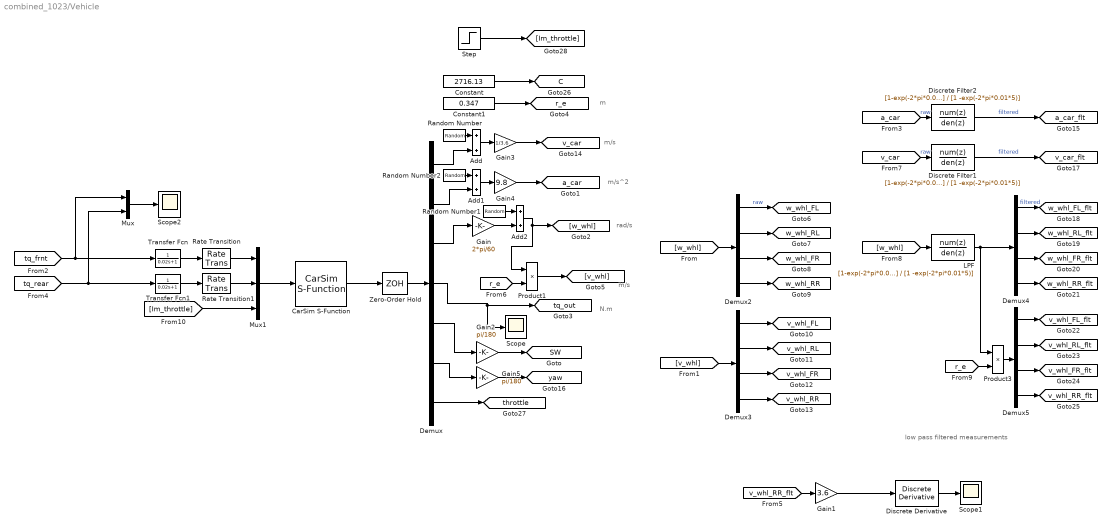
== system combined_1023/Vehicle ==
  note: low pass filtered measurements
  note: m/s
  note: m
  note: m/s
  note: rad/s
  note: N.m
  note: m/s^2
  Add : Sum
  Add1 : Sum
  Add2 : Sum
  CarSim S-Function : Solver_SF/CarSim S-Function  Priority=1  SIMFILE=simfile.sim  Run_RTs=off  vs_state_ind=Run  StopMode_ind=Vehicle Model
  Constant : Constant  Value=2716.13
  Constant1 : Constant  Value=0.347
  Demux : Demux  Outputs=[1 1 4 4 1 1 1]
  Demux{2..5} (4 alike) : Demux
  Discrete Derivative : simulink/Discrete/Discrete Derivative  gainval=1.0  ICPrevScaledInput=0.0  OutMin=[]  OutMax=[]  OutDataType=fixdt(1, 16)  OutScaling=2^-10  DoSatur=off
  Discrete Filter1 : DiscreteFilter  Numerator=[1-exp(-2*pi*0.01*5)]  Denominator=[1 -exp(-2*pi*0.01*5)]  SampleTime=0.01
  Discrete Filter2 : DiscreteFilter  Numerator=[1-exp(-2*pi*0.01*5)]  Denominator=[1 -exp(-2*pi*0.01*5)]  SampleTime=0.01
  Gain : Gain  Gain=2*pi/60
  Gain1 : Gain  Gain=3.6
  Gain2 : Gain  Gain=pi/180
  Gain3 : Gain  Gain=1/3.6
  Gain4 : Gain  Gain=9.8
  Gain5 : Gain  Gain=pi/180
  LPF : DiscreteFilter  Numerator=[1-exp(-2*pi*0.01*5)]  Denominator=[1 -exp(-2*pi*0.01*5)]  SampleTime=0.01
  Mux : Mux  Inputs=2
  Mux1 : Mux  Inputs=3
  Product1 : Product
  Product3 : Product
  Random Number : RandomNumber  Variance=0.0005  Seed=2  SampleTime=0.01
  Random Number1 : RandomNumber  Variance=0.002  Seed=2  SampleTime=0.01
  Random Number2 : RandomNumber  Variance=0.0002  Seed=2  SampleTime=0.01
  Rate Transition : RateTransition  OutPortSampleTime=0.01
  Rate Transition1 : RateTransition  OutPortSampleTime=0.01
  Scope : Scope
  Scope1 : Scope
  Scope2 : Scope
  Step : Step  Time=5  Before=0.2  After=0  SampleTime=0
  Transfer Fcn : TransferFcn  Denominator=[0.02 1]
  Transfer Fcn1 : TransferFcn  Denominator=[0.02 1]
  Zero-Order Hold : ZeroOrderHold  SampleTime=0.01
  tag scope: C=global, SW=global, a_car=global, a_car_flt=global, r_e=global, throttle=global, tq_out=global, v_car=global, v_car_flt=global, v_whl_FL=global, v_whl_FL_flt=global, v_whl_FR=global, v_whl_FR_flt=global, v_whl_RL=global, v_whl_RL_flt=global, v_whl_RR=global, v_whl_RR_flt=global, w_whl_FL=global, w_whl_FL_flt=global, w_whl_FR=global, w_whl_FR_flt=global, w_whl_RL=global, w_whl_RL_flt=global, w_whl_RR=global, w_whl_RR_flt=global, yaw=global
  wires:
  Constant1/1 -> [r_e]
  [r_e] -> Product1/2
  Product1/1 -> [v_whl]
  Demux3/4 -> [v_whl_RR]
  Demux3/2 -> [v_whl_RL]
  [v_whl] -> Demux3/1
  Demux3/1 -> [v_whl_FL]
  Demux3/3 -> [v_whl_FR]
  Gain/1 -> Add2/2
  Demux/2 -> Add1/2
  Demux/3 -> Gain/1
  Gain4/1 -> [a_car]
  Demux/4 -> Scope/1, [tq_out]
  CarSim S-Function/1 -> Zero-Order Hold/1
  Demux2/2 -> [w_whl_RL]
  Gain3/1 -> [v_car]
  Demux2/1 -> [w_whl_FL]  "raw"
  Demux/1 -> Add/2
  Demux2/3 -> [w_whl_FR]
  Zero-Order Hold/1 -> Demux/1
  [w_whl] -> Demux2/1
  Demux2/4 -> [w_whl_RR]
  Transfer Fcn/1 -> Rate Transition/1
  Transfer Fcn1/1 -> Rate Transition1/1
  Mux1/1 -> CarSim S-Function/1
  Rate Transition/1 -> Mux1/1
  Rate Transition1/1 -> Mux1/2
  [tq_frnt] -> Mux/1, Transfer Fcn/1
  [tq_rear] -> Mux/2, Transfer Fcn1/1
  Random Number/1 -> Add/1
  Add/1 -> Gain3/1
  Random Number2/1 -> Add1/1
  Add1/1 -> Gain4/1
  Random Number1/1 -> Add2/1
  Add2/1 -> Product1/1, [w_whl]
  [v_car] -> Discrete Filter1/1  "raw"
  Discrete Filter1/1 -> [v_car_flt]  "filtered"
  [w_whl] -> LPF/1
  LPF/1 -> Demux4/1, Product3/1
  Demux4/1 -> [w_whl_FL_flt]  "filtered"
  Demux4/2 -> [w_whl_RL_flt]
  Demux4/3 -> [w_whl_FR_flt]
  Demux4/4 -> [w_whl_RR_flt]
  [r_e] -> Product3/2
  Product3/1 -> Demux5/1
  Demux5/1 -> [v_whl_FL_flt]
  Demux5/2 -> [v_whl_RL_flt]
  Demux5/3 -> [v_whl_FR_flt]
  Demux5/4 -> [v_whl_RR_flt]
  [a_car] -> Discrete Filter2/1  "raw"
  Discrete Filter2/1 -> [a_car_flt]  "filtered"
  [v_whl_RR_flt] -> Gain1/1
  Discrete Derivative/1 -> Scope1/1
  Gain1/1 -> Discrete Derivative/1
  Demux/5 -> Gain2/1
  Demux/6 -> Gain5/1
  Gain2/1 -> [SW]
  Constant/1 -> [C]
  Gain5/1 -> [yaw]
  Demux/7 -> [throttle]
  Step/1 -> [Im_throttle]
  Mux/1 -> Scope2/1
  [Im_throttle] -> Mux1/3

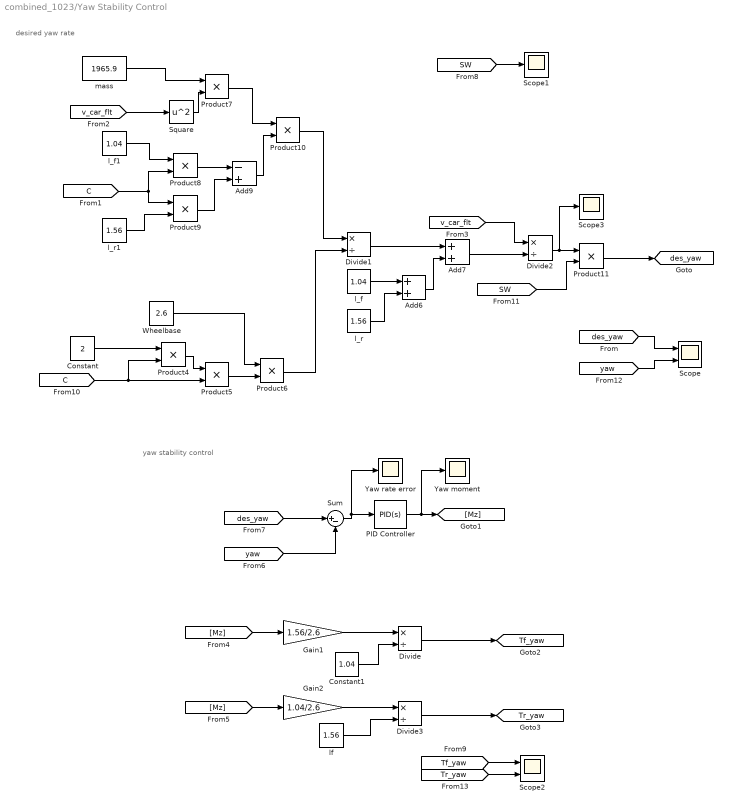
== system combined_1023/Yaw Stability Control ==
  note: yaw stability control
  note: desired yaw rate
  Add6 : Sum
  Add7 : Sum
  Add9 : Sum  Inputs=-+
  Constant : Constant  Value=2
  Constant1 : Constant  Value=1.04
  Divide{,1..3} (4 alike) : Product  Inputs=*/
  Gain1 : Gain  Gain=1.56/2.6
  Gain2 : Gain  Gain=1.04/2.6
  PID Controller : slpidlib/PID Controller  Controller=PID  Form=Parallel  TimeDomain=Continuous-time  UseExternalTs=off  SampleTime=-1  IntegratorMethod=Forward Euler  FilterMethod=Forward Euler  ControllerParametersSource=internal  P=180  I=0.001  UseKiTs=off  D=8  N=50  UseFilter=on  TunerSelectOption=Transfer Function Based (PID Tuner App)  InitialConditionSource=internal  InitialConditionForIntegrator=0  InitialConditionForFilter=0  DifferentiatorICPrevScaledInput=0  ExternalReset=none  TrackingMode=off  Kt=1  LimitOutput=off  SatLimitsSource=internal  UpperSaturationLimit=inf  LowerSaturationLimit=-inf  LinearizeAsGain=on  AntiWindupMode=none  Kb=1  LimitIntegrator=off  UpperIntegratorSaturationLimit=inf  LowerIntegratorSaturationLimit=-inf  POutMin=[]  POutMax=[]  IOutMin=[]  IOutMax=[]  DOutMin=[]  DOutMax=[]  NOutMin=[]  NOutMax=[]  SumOutMin=[]  SumOutMax=[]  SaturationOutMin=[]  SaturationOutMax=[]  PParamMin=[]  PParamMax=[]  IParamMin=[]  IParamMax=[]  DParamMin=[]  DParamMax=[]  NParamMin=[]  NParamMax=[]  KbParamMin=[]  KbParamMax=[]  KtParamMin=[]  KtParamMax=[]  KbOutMin=[]  KbOutMax=[]  KtOutMin=[]  KtOutMax=[]  IntegratorOutMin=[]  IntegratorOutMax=[]  FilterOutMin=[]  FilterOutMax=[]  SumI1OutMin=[]  SumI1OutMax=[]  SumI2OutMin=[]  SumI2OutMax=[]  SumI3OutMin=[]  SumI3OutMax=[]  SumI4OutMin=[]  SumI4OutMax=[]  SumDOutMin=[]  SumDOutMax=[]  DifferentiatorOutMin=[]  DifferentiatorOutMax=[]  FilterDiffOutCoefMin=[]  FilterDiffOutCoefMax=[]  ReciprocalOutMin=[]  ReciprocalOutMax=[]  SumDenOutMin=[]  SumDenOutMax=[]  SumNumOutMin=[]  SumNumOutMax=[]  DivideOutMin=[]  DivideOutMax=[]  UdiffTsProdOutMin=[]  UdiffTsProdOutMax=[]  NTsProdOutMin=[]  NTsProdOutMax=[]  UintegralTsProdOutMin=[]  UintegralTsProdOutMax=[]  UngainTsProdOutMin=[]  UngainTsProdOutMax=[]  ClampingZeroOutDataTypeStr=Inherit: Inherit via back propagation  ClampingZeroOutMin=[]  ClampingZeroOutMax=[]  FilterDenConstantOutDataTypeStr=Inherit: Inherit via back propagation  FilterDenConstantOutMin=[]  FilterDenConstantOutMax=[]  PCopyOutDataTypeStr=Inherit: Inherit via back propagation  PCopyOutMin=[]  PCopyOutMax=[]  NCopyOutDataTypeStr=Inherit: Inherit via back propagation  NCopyOutMin=[]  NCopyOutMax=[]  IntegratorContinuousStateAttributes=''  IntegratorStateMustResolveToSignalObject=off  IntegratorRTWStateStorageClass=Auto  FilterContinuousStateAttributes=''  FilterStateMustResolveToSignalObject=off  FilterRTWStateStorageClass=Auto  ParallelPVariant=InternalParameters  IdealPVariant=Disabled  IVariant=InternalParameters  DVariant=InternalParameters  IntegratorVariant=Continuous  SatVariant=Disabled  AWVariant=Passthrough  PCopyVariant=Disabled  TRVariant=Disabled  FdbkBlocksVariant=Forward  IdealPFdbkVariant=Disabled  SatFdbkVariant=Disabled  DerivativeFilterVariant=ContFilter  NVariant=InternalParameters  NCopyVariant=Disabled  FilterICVariant=InternalICsFilter  IntegratorICVariant=InternalICs  ExternalResetVariant=Disabled  TRSumVariant=Passthrough  SumFdbkVariant=Disabled  SumVariant=Sum_PID  TsampFilterVariant=InternalTs  TsampNgainVariant=Passthrough  TsampIntegralVariant=Disabled_SignalSpec  ExternalSaturationOutDataTypeStr=Inherit: Same as second input
  Product{4..11} (8 alike) : Product
  Scope : Scope  NumInputPorts=2
  Scope1 : Scope
  Scope2 : Scope  NumInputPorts=2
  Scope3 : Scope
  Square : Math  Operator=square
  Sum : Sum  Inputs=|+-
  Wheelbase : Constant  Value=2.6
  Yaw moment : Scope
  Yaw rate error : Scope
  l_f : Constant  Value=1.04
  l_f1 : Constant  Value=1.04
  l_r : Constant  Value=1.56
  l_r1 : Constant  Value=1.56
  lf : Constant  Value=1.56
  mass : Constant  Value=1965.9
  tag scope: Tf_yaw=global, Tr_yaw=global, des_yaw=global
  wires:
  Add9/1 -> Product10/2
  Add6/1 -> Add7/2
  l_r/1 -> Add6/2
  Product11/1 -> [des_yaw]
  Square/1 -> Product7/2
  l_f/1 -> Add6/1
  Product6/1 -> Divide1/2
  Product7/1 -> Product10/1
  Product4/1 -> Product5/1
  Product5/1 -> Product6/2
  Divide2/1 -> Scope3/1, Product11/1
  l_r1/1 -> Product9/2
  [v_car_flt] -> Divide2/1
  Product8/1 -> Add9/1
  [v_car_flt] -> Square/1
  l_f1/1 -> Product8/1
  [C] -> Product5/2, Product4/2
  Product10/1 -> Divide1/1
  Divide1/1 -> Add7/1
  Wheelbase/1 -> Product6/1
  Constant/1 -> Product4/1
  [C] -> Product9/1, Product8/2
  Add7/1 -> Divide2/2
  mass/1 -> Product7/1
  [SW] -> Product11/2
  [des_yaw] -> Scope/1
  [yaw] -> Scope/2
  Product9/1 -> Add9/2
  [yaw] -> Sum/2
  [des_yaw] -> Sum/1
  Divide/1 -> [Tf_yaw]
  lf/1 -> Divide3/2
  Divide3/1 -> [Tr_yaw]
  Constant1/1 -> Divide/2
  PID Controller/1 -> Yaw moment/1, [Mz]
  [Mz] -> Gain2/1
  [Mz] -> Gain1/1
  Gain2/1 -> Divide3/1
  Sum/1 -> PID Controller/1, Yaw rate error/1
  Gain1/1 -> Divide/1
  [SW] -> Scope1/1
  [Tf_yaw] -> Scope2/1
  [Tr_yaw] -> Scope2/2

== system combined_1023/Coasting Torque Command/If Action Subsystem ==
  Action Port : ActionPort  ActionPortLabel=if(u1 < 0 & u2 < 0)
  Constant : Constant  SampleTime=0.01
  flag : Outport
  wires:
  Constant/1 -> flag/1

== system combined_1023/Coasting Torque Command/If Action Subsystem1 ==
  Action Port : ActionPort  ActionPortLabel=else
  Constant : Constant  Value=0  SampleTime=0.01
  flag : Outport
  wires:
  Constant/1 -> flag/1

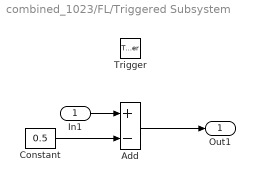
== system combined_1023/FL/Triggered Subsystem ==
  In1 : Inport
  Trigger : TriggerPort  VariantControl=(inherit)
  Add : Sum  Inputs=+-
  Constant : Constant  Value=0.5
  Out1 : Outport
  wires:
  In1/1 -> Add/1
  Constant/1 -> Add/2
  Add/1 -> Out1/1

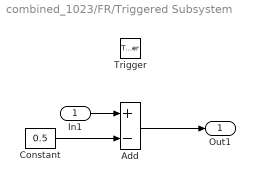
== system combined_1023/FR/Triggered Subsystem ==
  In1 : Inport
  Trigger : TriggerPort  VariantControl=(inherit)
  Add : Sum  Inputs=+-
  Constant : Constant  Value=0.5
  Out1 : Outport
  wires:
  In1/1 -> Add/1
  Constant/1 -> Add/2
  Add/1 -> Out1/1

== system combined_1023/RL/Triggered Subsystem ==
  In1 : Inport
  Trigger : TriggerPort  VariantControl=(inherit)
  Add : Sum  Inputs=+-
  Constant : Constant  Value=0.5
  Out1 : Outport
  wires:
  Add/1 -> Out1/1
  Constant/1 -> Add/2
  In1/1 -> Add/1

== system combined_1023/RR/Triggered Subsystem ==
  In1 : Inport
  Trigger : TriggerPort  VariantControl=(inherit)
  Add : Sum  Inputs=+-
  Constant : Constant  Value=0.5
  Out1 : Outport
  wires:
  In1/1 -> Add/1
  Constant/1 -> Add/2
  Add/1 -> Out1/1

== stateflow chart combined_1023/RR/Chart1 ==
  state LSC_On
    state Phase7
      entry,during:
      phase = 7;
    state Phase6
      entry,during:
      phase = 6;
    state Phase1
      entry,during:
      phase = 1;
    state Phase2
      entry,during:
      phase = 2;
    state Phase3
      entry,during:
      phase = 3;
    state Phase4
      entry,during:
      phase = 4;
    state Phase5
      entry,during:
      phase = 5;
    Phase7 -> (junction 235) [order 2] : [(slip > 0.95*slip_max)]
    (junction 235) -> (junction 167)
    Phase6 -> Phase7 [order 2] : [(slip > 0.85*slip_max)]
    Phase7 -> Phase6 [order 1] : [(slip_pred < slip_max)]
    Phase6 -> (junction 225) [order 1] : [(tq_cmd < tq_in)&(slip < 0.5*slip_max)]
    (junction 225) -> Phase1
    Phase2 -> Phase6 [order 1] : [(slip_pred < 0.85*slip_max)]
    (default) -> Phase1
    Phase1 -> Phase2 : [(slip_pred > 0.95*slip_max)]
    (junction 167) -> Phase2
    (junction 165) -> (junction 167)
    (junction 217) -> Phase1
    Phase2 -> Phase3 [order 2] : [(slip > 0.9*slip_max)]
    Phase3 -> Phase4 : [(slip_pred < slip_max)]
    Phase4 -> (junction 217) [order 1] : [(tq_cmd < tq_in)]
    (junction 220) -> (junction 217)
    Phase4 -> Phase5 [order 2] : [(a_whl < 0)]
    Phase5 -> (junction 220) [order 1] : [(tq_cmd < tq_in)]
    Phase5 -> (junction 165) [order 2] : [(slip_pred > slip_max)]
  state LSC_off
    entry,during:
    phase = 0;
  state ready
    phase = 0;
  LSC_On -> (junction 231) : [(coast_flag ~= 1)]
  (junction 231) -> ready
  (default) -> ready
  LSC_off -> LSC_On : [(a_whl < 0)&(slip > 0)&(a_car < 0)]
  ready -> LSC_off : [(coast_flag == 1)]
  data: a_whl input; phase output; slip input; a_car input; coast_flag input; slip_pred input; slip_max input; tq_cmd input; tq_in input

== stateflow chart combined_1023/RL/Chart1 ==
  state LSC_On
    state Phase7
      entry,during:
      phase = 7;
    state Phase6
      entry,during:
      phase = 6;
    state Phase1
      entry,during:
      phase = 1;
    state Phase2
      entry,during:
      phase = 2;
    state Phase3
      entry,during:
      phase = 3;
    state Phase4
      entry,during:
      phase = 4;
    state Phase5
      entry,during:
      phase = 5;
    Phase7 -> (junction 235) [order 2] : [(slip > 0.95*slip_max)]
    (junction 235) -> (junction 167)
    Phase6 -> Phase7 [order 2] : [(slip > 0.85*slip_max)]
    Phase7 -> Phase6 [order 1] : [(slip_pred < slip_max)]
    Phase6 -> (junction 225) [order 1] : [(tq_cmd < tq_in)&(slip < 0.5*slip_max)]
    (junction 225) -> Phase1
    Phase2 -> Phase6 [order 1] : [(slip_pred < 0.85*slip_max)]
    (default) -> Phase1
    Phase1 -> Phase2 : [(slip_pred > 0.95*slip_max)]
    (junction 167) -> Phase2
    (junction 165) -> (junction 167)
    (junction 217) -> Phase1
    Phase2 -> Phase3 [order 2] : [(slip > 0.9*slip_max)]
    Phase3 -> Phase4 : [(slip_pred < slip_max)]
    Phase4 -> (junction 217) [order 1] : [(tq_cmd < tq_in)]
    (junction 220) -> (junction 217)
    Phase4 -> Phase5 [order 2] : [(a_whl < 0)]
    Phase5 -> (junction 220) [order 1] : [(tq_cmd < tq_in)]
    Phase5 -> (junction 165) [order 2] : [(slip_pred > slip_max)]
  state LSC_off
    entry,during:
    phase = 0;
  state ready
    phase = 0;
  LSC_On -> (junction 231) : [(coast_flag ~= 1)]
  (junction 231) -> ready
  (default) -> ready
  LSC_off -> LSC_On : [(a_whl < 0)&&(slip > 0)&&(a_car < 0)]
  ready -> LSC_off : [(coast_flag == 1)]
  data: a_whl input; phase output; slip input; a_car input; coast_flag input; slip_pred input; slip_max input; tq_cmd input; tq_in input

== stateflow chart combined_1023/FR/Chart1 ==
  state LSC_On
    state Phase7
      entry,during:
      phase = 7;
    state Phase6
      entry,during:
      phase = 6;
    state Phase1
      entry,during:
      phase = 1;
    state Phase2
      entry,during:
      phase = 2;
    state Phase3
      entry,during:
      phase = 3;
    state Phase4
      entry,during:
      phase = 4;
    state Phase5
      entry,during:
      phase = 5;
    Phase7 -> (junction 235) [order 2] : [(slip > 0.95*slip_max)]
    (junction 235) -> (junction 167)
    Phase6 -> Phase7 [order 2] : [(slip > 0.85*slip_max)]
    Phase7 -> Phase6 [order 1] : [(slip_pred < slip_max)]
    Phase6 -> (junction 225) [order 1] : [(tq_cmd < tq_in)&(slip < 0.5*slip_max)]
    (junction 225) -> Phase1
    Phase2 -> Phase6 [order 1] : [(slip_pred < 0.85*slip_max)]
    (default) -> Phase1
    Phase1 -> Phase2 : [(slip_pred > 0.95*slip_max)]
    (junction 167) -> Phase2
    (junction 165) -> (junction 167)
    (junction 217) -> Phase1
    Phase2 -> Phase3 [order 2] : [(slip > 0.9*slip_max)]
    Phase3 -> Phase4 : [(slip_pred < slip_max)]
    Phase4 -> (junction 217) [order 1] : [(tq_cmd < tq_in)]
    (junction 220) -> (junction 217)
    Phase4 -> Phase5 [order 2] : [(a_whl < 0)]
    Phase5 -> (junction 220) [order 1] : [(tq_cmd < tq_in)]
    Phase5 -> (junction 165) [order 2] : [(slip_pred > slip_max)]
  state LSC_off
    entry,during:
    phase = 0;
  state ready
    phase = 0;
  LSC_On -> (junction 231) : [(coast_flag ~= 1)]
  (junction 231) -> ready
  (default) -> ready
  LSC_off -> LSC_On : [(a_whl < 0)&&(slip > 0)&&(a_car < 0)]
  ready -> LSC_off : [(coast_flag == 1)]
  data: a_whl input; phase output; slip input; a_car input; coast_flag input; slip_pred input; slip_max input; tq_cmd input; tq_in input

== stateflow chart combined_1023/FL/Chart1 ==
  state LSC_On
    state Phase7
      entry,during:
      phase = 7;
    state Phase6
      entry,during:
      phase = 6;
    state Phase1
      entry,during:
      phase = 1;
    state Phase2
      entry,during:
      phase = 2;
    state Phase3
      entry,during:
      phase = 3;
    state Phase4
      entry,during:
      phase = 4;
    state Phase5
      entry,during:
      phase = 5;
    Phase7 -> (junction 235) [order 2] : [(slip > 0.95*slip_max)]
    (junction 235) -> (junction 167)
    Phase6 -> Phase7 [order 2] : [(slip > 0.85*slip_max)]
    Phase7 -> Phase6 [order 1] : [(slip_pred < slip_max)]
    Phase6 -> (junction 225) [order 1] : [(tq_cmd < tq_in)&(slip < 0.5*slip_max)]
    (junction 225) -> Phase1
    Phase2 -> Phase6 [order 1] : [(slip_pred < 0.85*slip_max)]
    (default) -> Phase1
    Phase1 -> Phase2 : [(slip_pred > 0.95*slip_max)]
    (junction 167) -> Phase2
    (junction 165) -> (junction 167)
    (junction 217) -> Phase1
    Phase2 -> Phase3 [order 2] : [(slip > 0.9*slip_max)]
    Phase3 -> Phase4 : [(slip_pred < slip_max)]
    Phase4 -> (junction 217) [order 1] : [(tq_cmd < tq_in)]
    (junction 220) -> (junction 217)
    Phase4 -> Phase5 [order 2] : [(a_whl < 0)]
    Phase5 -> (junction 220) [order 1] : [(tq_cmd < tq_in)]
    Phase5 -> (junction 165) [order 2] : [(slip_pred > slip_max)]
  state LSC_off
    entry,during:
    phase = 0;
  state ready
    phase = 0;
  LSC_On -> (junction 231) : [(coast_flag ~= 1)]
  (junction 231) -> ready
  (default) -> ready
  LSC_off -> LSC_On : [(a_whl < 0)&&(slip > 0)&&(a_car < 0)]
  ready -> LSC_off : [(coast_flag == 1)]
  data: a_whl input; phase output; slip input; a_car input; coast_flag input; slip_pred input; slip_max input; tq_cmd input; tq_in input

== stateflow chart combined_1023/Coasting Torque Command/Slip Stateflow ==
  state Coasting
    state State0
      state = 0;
    state State1
      "No Slip"
      state = 1;
    state State2
      "Frnt Slip"
      state = 2;
    state State3
      "Rear Slip"
      state = 3;
    state State4
      "Both Slip"
      state = 4;
    (default) -> State0
    State0 -> State1 : [(ph_FL==1)&(ph_FR==1)&(ph_RL==1)&(ph_RR==1)&(SW>=0.05)]
    State1 -> State2 [order 1] : [(ph_FL~=1)|(ph_FR~=1)]
    State2 -> State1 [order 1] : [(ph_FL==1)&(ph_FR==1)]
    State3 -> State1 [order 1] : [(ph_RL==1)&(ph_RR==1)]
    State1 -> State3 [order 2] : [(ph_RL~=1)|(ph_RR~=1)]
    State4 -> State2 [order 1] : [(ph_RL==1)&(ph_RR==1)]
    State2 -> State4 [order 2] : [(ph_RL~=1)|(ph_RR~=1)]
    State3 -> State4 [order 2] : [(ph_FL~=1)|(ph_FR~=1)]
    State4 -> State3 [order 2] : [(ph_FL==1)&(ph_FR==1)]
  state drive
    state = 0;
  Coasting -> (junction 33) : [(coast_flag ~= 1)&(throttle > 0.05)]
  (junction 33) -> drive
  (default) -> drive
  drive -> Coasting : [(coast_flag == 1)&(throttle <= 0.05)]
  data: coast_flag input; ph_FL input; ph_FR input; ph_RL input; ph_RR input; state output; SW input; throttle input
